simulink model "dc_microgrid_vreg"  (R2015a)
settings: Solver=ode45  StartTime=0.0  StopTime=0.01  RelTol=1e-3
values from neighbouring files (symbols this model uses):
  A = 25*[0 1;1 0]    [parameters_dcmicrogrid.m]    (also in parameters_dcmicrogrid_hynger.m; pendulum_init.m = [0 1 0 0)
  a1v1 = Pmc*a1xpi1    [parameters_dcmicrogrid.m]    (also in parameters_dcmicrogrid_hynger.m)
  a1v2 = Pmc*a1xpi2    [parameters_dcmicrogrid.m]    (also in parameters_dcmicrogrid_hynger.m)
  a1xmc1 = a3    [parameters_dcmicrogrid.m]    (also in parameters_dcmicrogrid_hynger.m)
  a1xmc2 = a3    [parameters_dcmicrogrid.m]    (also in parameters_dcmicrogrid_hynger.m)
  a1xpi1 = Imc*c3    [parameters_dcmicrogrid.m]    (also in parameters_dcmicrogrid_hynger.m)
  a1xpi2 = Imc*c3    [parameters_dcmicrogrid.m]    (also in parameters_dcmicrogrid_hynger.m)
  a2v1 = Pmc*a2xpi1    [parameters_dcmicrogrid.m]    (also in parameters_dcmicrogrid_hynger.m)
  a2v2 = Pmc*a2xpi2    [parameters_dcmicrogrid.m]    (also in parameters_dcmicrogrid_hynger.m)
  a2xmc1 = C(1,2)*P(1,1)*c1/Imax(1)    [parameters_dcmicrogrid.m]    (also in parameters_dcmicrogrid_hynger.m)
  a2xmc2 = C(2,1)*P(2,2)*c1/Imax(2)    [parameters_dcmicrogrid.m]    (also in parameters_dcmicrogrid_hynger.m)
  a2xpi1 = Imc*c2    [parameters_dcmicrogrid.m]    (also in parameters_dcmicrogrid_hynger.m)
  a2xpi2 = Imc*c2    [parameters_dcmicrogrid.m]    (also in parameters_dcmicrogrid_hynger.m)
  a3xmc1 = C(1,2)*P(1,1)*c1/Imax(1) + RD(1,1)*c1    [parameters_dcmicrogrid.m]    (also in parameters_dcmicrogrid_hynger.m)
  a3xmc2 = C(1,2)*P(2,2)*c1/Imax(2) + RD(2,2)*c1    [parameters_dcmicrogrid.m]    (also in parameters_dcmicrogrid_hynger.m)
  axi1 = C(1,2)*I(1,1)*c1/Imax(1)    [parameters_dcmicrogrid.m]    (also in parameters_dcmicrogrid_hynger.m)
  axi2 = C(2,1)*I(2,2)*c1/Imax(2)    [parameters_dcmicrogrid.m]    (also in parameters_dcmicrogrid_hynger.m)
  B = 1*A    [parameters_dcmicrogrid.m]    (also in parameters_dcmicrogrid_hynger.m; pendulum_init.m = [0 ; 1.94 ; 0 ; -4.44 ])
  b2 = 1.94    [pendulum_init.m]
  C1 = 2.2e-3    (= 0.0022)    [parameters_dcmicrogrid.m]    (also in parameters_dcmicrogrid_hynger.m)
  C2 = 2.2e-3    (= 0.0022)    [parameters_dcmicrogrid.m]    (also in parameters_dcmicrogrid_hynger.m)
  I = 3*[1 0; 0 1]    [parameters_dcmicrogrid.m]    (also in parameters_dcmicrogrid_hynger.m)
  iL1_0 = 3.2    [parameters_dcmicrogrid_hynger.m]
  iL2_0 = 3.2    [parameters_dcmicrogrid_hynger.m]
  K = [1 0; 0 2]    [parameters_dcmicrogrid_hynger.m]    (also in pendulum_init.m = K_lmi)
  L1 = 2.65e-3    (= 0.00265)    [parameters_dcmicrogrid.m]    (also in parameters_dcmicrogrid_hynger.m)
  L2 = 2.65e-3    (= 0.00265)    [parameters_dcmicrogrid.m]    (also in parameters_dcmicrogrid_hynger.m)
  P = 0.05*[1 0; 0 1]    [parameters_dcmicrogrid.m]    (also in parameters_dcmicrogrid_hynger.m; pendulum_init.m = [p11 p12 p13 p14; p12 p22 p23 p24; p13 p23 p33 p34; p14 p24 )
  R1 = 20    [parameters_dcmicrogrid.m]    (also in parameters_dcmicrogrid_hynger.m = 30)
  R2 = 20    [parameters_dcmicrogrid.m]    (also in parameters_dcmicrogrid_hynger.m = 30)
  Req = R1*R2/(R1+R2)    (= 10)    [parameters_dcmicrogrid.m]    (also in parameters_dcmicrogrid_hynger.m = 15)
  rL1 = 520e-3    (= 0.52)    [parameters_dcmicrogrid.m]    (also in parameters_dcmicrogrid_hynger.m)
  rL2 = 520e-3    (= 0.52)    [parameters_dcmicrogrid.m]    (also in parameters_dcmicrogrid_hynger.m)
  rs1 = 200e-3    (= 0.2)    [parameters_dcmicrogrid.m]    (also in parameters_dcmicrogrid_hynger.m)
  rs2 = 200e-3    (= 0.2)    [parameters_dcmicrogrid.m]    (also in parameters_dcmicrogrid_hynger.m)
  T1 = 1/60000    (= 1.66666666667e-05)    [parameters_dcmicrogrid.m]    (also in parameters_dcmicrogrid_hynger.m = 6.66666666667e-05)
  T2 = 1/60000    (= 1.66666666667e-05)    [parameters_dcmicrogrid.m]    (also in parameters_dcmicrogrid_hynger.m = 6.66666666667e-05)
  t_0 = 0    [parameters_dcmicrogrid_hynger.m]
  vavgi1_0 = 0    [parameters_dcmicrogrid_hynger.m]
  vavgi2_0 = 0    [parameters_dcmicrogrid_hynger.m]
  vC1_0 = 48.02    [parameters_dcmicrogrid_hynger.m]
  vC2_0 = 48.02    [parameters_dcmicrogrid_hynger.m]
  vesti1_0 = 48.02    [parameters_dcmicrogrid_hynger.m]
  vesti2_0 = 48.02    [parameters_dcmicrogrid_hynger.m]
  Vin1 = Vin(1)    [parameters_dcmicrogrid.m]    (also in parameters_dcmicrogrid_hynger.m)
  Vin2 = Vin(2)    [parameters_dcmicrogrid.m]    (also in parameters_dcmicrogrid_hynger.m)
  Vref1 = Vref(1)    [parameters_dcmicrogrid.m]    (also in parameters_dcmicrogrid_hynger.m)
  Vref2 = Vref(2)    [parameters_dcmicrogrid.m]    (also in parameters_dcmicrogrid_hynger.m)
  westi1_0 = 0    [parameters_dcmicrogrid_hynger.m]
  westi2_0 = 0    [parameters_dcmicrogrid_hynger.m]
  westii1_0 = 0    [parameters_dcmicrogrid_hynger.m]
  westii2_0 = 0    [parameters_dcmicrogrid_hynger.m]
  xi1_0 = 0.01915    [parameters_dcmicrogrid_hynger.m]
  xi2_0 = 0.01915    [parameters_dcmicrogrid_hynger.m]
  xmc1_0 = 2.401    [parameters_dcmicrogrid_hynger.m]
  xmc2_0 = 2.401    [parameters_dcmicrogrid_hynger.m]
  xpi1_0 = 0.51    [parameters_dcmicrogrid_hynger.m]
  xpi2_0 = 0.51    [parameters_dcmicrogrid_hynger.m]
  xpu1_0 = 0.008491    [parameters_dcmicrogrid_hynger.m]
  xpu2_0 = 0.008491    [parameters_dcmicrogrid_hynger.m]
  xvo1_0 = 0.0103    [parameters_dcmicrogrid_hynger.m]
  xvo2_0 = 0.0103    [parameters_dcmicrogrid_hynger.m]
undefined symbols (not defined in the file or in its folder): a1, a2, b1, c1, c2, d1, d2
settings Model: CovSFcnEnable=off  Creator=OmarAli  LastModifiedBy=omar
settings DataIOCC: LimitDataPoints=off
settings DebuggingCC: SolverPrmCheckMsg=warning

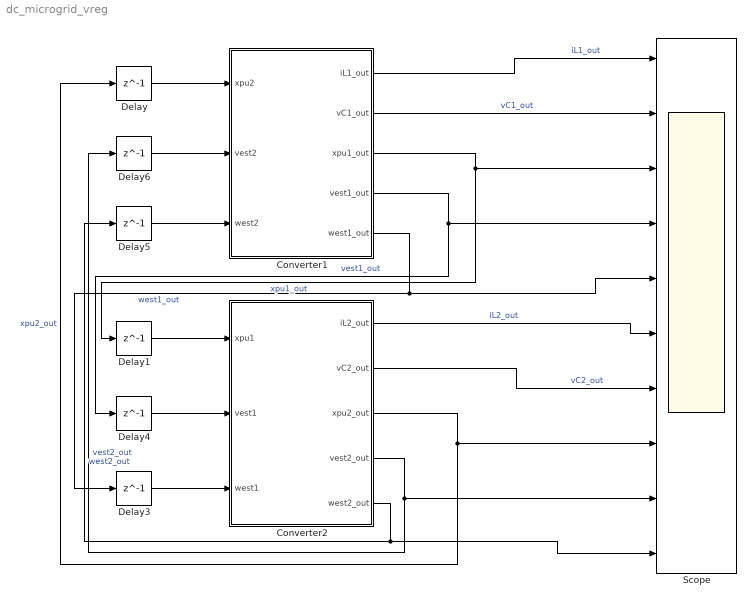
== system dc_microgrid_vreg ==
  Converter1 : Stateflow chart  TreatAsAtomicUnit=on
  Converter2 : Stateflow chart  TreatAsAtomicUnit=on
  Delay{,1,3..6} (6 alike) : Delay  DelayLength=1  InitialCondition=0  SampleTime=1/60000
  Scope : Scope  NumInputPorts=10
      settings: ShowLegends=on  YMin=0~0~0~0~-0.0125~0~0~0~0~-0.0125  YMax=2.5~20~0.0075~20~0.0025~2.5~20~0.0075~20~0.0025
  wires:
  Converter1/3(xpu1_out) -> Scope/3, Delay1/1  "xpu1_out"
  Converter2/3(xpu2_out) -> Scope/8, Delay/1  "xpu2_out"
  Delay/1 -> Converter1/1(xpu2)
  Delay1/1 -> Converter2/1(xpu1)
  Converter1/1(iL1_out) -> Scope/1  "iL1_out"
  Converter1/2(vC1_out) -> Scope/2  "vC1_out"
  Delay4/1 -> Converter2/2(vest1)
  Delay3/1 -> Converter2/3(west1)
  Delay6/1 -> Converter1/2(vest2)
  Delay5/1 -> Converter1/3(west2)
  Converter2/5(west2_out) -> Scope/10, Delay5/1  "west2_out"
  Converter2/4(vest2_out) -> Scope/9, Delay6/1  "vest2_out"
  Converter1/4(vest1_out) -> Scope/4, Delay4/1  "vest1_out"
  Converter1/5(west1_out) -> Delay3/1, Scope/5  "west1_out"
  Converter2/1(iL2_out) -> Scope/6  "iL2_out"
  Converter2/2(vC2_out) -> Scope/7  "vC2_out"

== stateflow chart dc_microgrid_vreg/Converter2 ==
  settings: updateMethod=CONTINUOUS
  state close2
    du:
    iL2_dot = (1/L2)*(-1*(rs2+rL2)*iL2+Vin2 - vC2);
    vC2_dot = (1/C2)*(iL2 - vC2/R2);
    xpu2_dot = a1*xpu2 + b1*iL2;
    xi2_dot = axi2*(xpu1 - xpu2);
    xmc2_dot = a1xmc2*xmc2 + a2xmc2*xpu1 - a3xmc2*xpu2 + xi2+ Vref2+ vavgi2 + (Vref2 - vesti2 - a2xpi2*xvo2 + westii2*K(2,2))*P(2,2);
    xvo2_dot = a2*xvo2 + b2*vC2;
    xpi2_dot = a1xpi2*xmc2 - a2xpi2*xvo2;
    vesti2_dot = (vest1 - vesti2 - a2xpi2*xvo2+ westii2*K(2,2))*A(2,1);
    westi2_dot = (west1 - vesti2 + westii2*K(2,2) - westi2)*B(2,1);
    westii2_dot = vesti2 - westii2*K(2,2) + westi2;
    vavgi2_dot = (Vref2 - vesti2 -  a2xpi2*xvo2 +westii2*K(2,2))*I(2,2);
    t_dot = 1;
    iL2_out = iL2;
    vC2_out = vC2;
    xpu2_out = xpu2;
    vest2_out = vesti2 + a2xpi2*xvo2 - westii2*K(2,2);
    west2_out = westi2 + vesti2 - westii2*K(2,2);
  state open2
    du:
    iL2_dot = (1/L2)*(-rL2*iL2 - vC2);
    vC2_dot = (1/C2)*(iL2 - vC2/R2);
    xpu2_dot = a1*xpu2 + b1*iL2;
    xi2_dot = axi2*(xpu1 - xpu2);
    xmc2_dot = a1xmc2*xmc2 + a2xmc2*xpu1 - a3xmc2*xpu2 + xi2+ Vref2+ vavgi2 + (Vref2 - vesti2 - a2xpi2*xvo2 + westii2*K(2,2))*P(2,2);
    xvo2_dot = a2*xvo2 + b2*vC2;
    xpi2_dot = a1xpi2*xmc2 - a2xpi2*xvo2;
    vesti2_dot = (vest1 - vesti2 - a2xpi2*xvo2+ westii2*K(2,2))*A(2,1);
    westi2_dot = (west1 - vesti2 + westii2*K(2,2) - westi2)*B(2,1);
    westii2_dot = vesti2 - westii2*K(2,2) + westi2;
    vavgi2_dot = (Vref2 - vesti2 -  a2xpi2*xvo2 +westii2*K(2,2))*I(2,2);
    t_dot = 1;
    iL2_out = iL2;
    vC2_out = vC2;
    xpu2_out = xpu2;
    vest2_out = vesti2 + a2xpi2*xvo2 - westii2*K(2,2);
    west2_out = westi2 + vesti2 - westii2*K(2,2);
  state dcm2
    du:
    iL2_dot = 0;
    vC2_dot = - vC2/(R2*C2);
    xpu2_dot = a1*xpu2 + b1*iL2;
    xi2_dot = axi2*(xpu1 - xpu2);
    xmc2_dot = a1xmc2*xmc2 + a2xmc2*xpu1 - a3xmc2*xpu2 + xi2+ Vref2+ vavgi2 + (Vref2 - vesti2 - a2xpi2*xvo2 + westii2*K(2,2))*P(2,2);
    xvo2_dot = a2*xvo2 + b2*vC2;
    xpi2_dot = a1xpi2*xmc2 - a2xpi2*xvo2;
    vesti2_dot = (vest1 - vesti2 - a2xpi2*xvo2+ westii2*K(2,2))*A(2,1);
    westi2_dot = (west1 - vesti2 + westii2*K(2,2) - westi2)*B(2,1);
    westii2_dot = vesti2 - westii2*K(2,2) + westi2;
    vavgi2_dot = (Vref2 - vesti2 -  a2xpi2*xvo2 +westii2*K(2,2))*I(2,2);
    t_dot = 1;
    iL2_out = iL2;
    vC2_out = vC2;
    xpu2_out = xpu2;
    vest2_out = vesti2 + a2xpi2*xvo2 - westii2*K(2,2);
    west2_out = westi2 + vesti2 - westii2*K(2,2);
  close2 -> open2 : [(a1v2*xmc2 - a2v2*xvo2 + xpi2) -  t/T2<= 0]
  (default) -> close2 : {iL2 = iL2_0;
      | vC2 = vC2_0;
      | xpu2 = xpu2_0;
      | xi2 = xi2_0;
      | xmc2 = xmc2_0;
      | xvo2 = xvo2_0;
      | xpi2 = xpi2_0;
      | vesti2 = vesti2_0;
      | westi2 = westi2_0;
      | westii2 = westii2_0;
      | vavgi2 = vavgi2_0;
      | t = t_0;}
  open2 -> close2 [order 2] : [t >= T2]
      | {t = 0;}
  open2 -> dcm2 [order 1] : [iL2 <= 0]
  dcm2 -> close2 : [t >= T2]
      | {t = 0;}
  data: rs2 parameter double; Vref2 parameter double; Vin2 parameter double; rL2 parameter double; iL2_out output double; t local; iL2 local; vC2 local; xi2 local; xvo2 local; xpu2 local; xmc2 local; xpi2 local; T2 parameter double; L2 parameter double; C2 parameter double; R2 parameter double; vC2_out output double; xpu2_out output double; xpu1 input double; a1 parameter double; a2 parameter double; b1 parameter double; b2 parameter double; c1 parameter double; c2 parameter double; d1 parameter double; d2 parameter double; axi2 parameter double; a1xmc2 parameter double; a2xmc2 parameter double; a3xmc2 parameter double; a1xpi2 parameter double; a2xpi2 parameter double; a1v2 parameter double; a2v2 parameter double; Req parameter double; iL2_0 parameter; t_0 parameter; xpu2_0 parameter; xmc2_0 parameter; xvo2_0 parameter; xpi2_0 parameter; vC2_0 parameter; xi2_0 parameter; vest1 input double; west1 input double; vesti2_0 parameter; westi2_0 parameter; westii2_0 parameter; vavgi2_0 parameter; vest2_out output; west2_out output; westi2 local; vavgi2 local; vesti2 local; westii2 local; B parameter; I parameter; A parameter; P parameter; K parameter
  data t settings: updateMethod=SF_CONTINUOUS_TIME_DATA
  data iL2 settings: updateMethod=SF_CONTINUOUS_TIME_DATA
  data vC2 settings: updateMethod=SF_CONTINUOUS_TIME_DATA
  data xi2 settings: updateMethod=SF_CONTINUOUS_TIME_DATA
  data xvo2 settings: updateMethod=SF_CONTINUOUS_TIME_DATA
  data xpu2 settings: updateMethod=SF_CONTINUOUS_TIME_DATA
  data xmc2 settings: updateMethod=SF_CONTINUOUS_TIME_DATA
  data xpi2 settings: updateMethod=SF_CONTINUOUS_TIME_DATA
  data westi2 settings: updateMethod=SF_CONTINUOUS_TIME_DATA
  data vavgi2 settings: updateMethod=SF_CONTINUOUS_TIME_DATA
  data vesti2 settings: updateMethod=SF_CONTINUOUS_TIME_DATA
  data westii2 settings: updateMethod=SF_CONTINUOUS_TIME_DATA

== stateflow chart dc_microgrid_vreg/Converter1 ==
  settings: updateMethod=CONTINUOUS
  state open1
    du:
    iL1_dot = (1/L1)*(-rL1*iL1 - vC1);
    vC1_dot = (1/C1)*(iL1 - vC1/R1);
    xpu1_dot = a1*xpu1 + b1*iL1;
    xi1_dot = axi1*(xpu2 - xpu1);
    xmc1_dot = a1xmc1*xmc1 + a2xmc1*xpu2  - a3xmc1*xpu1 + xi1+ Vref1+ vavgi1 + (Vref1 - vesti1 - a2xpi1*xvo1 + westii1*K(1,1))*P(1,1);
    xvo1_dot = a2*xvo1 + b2*vC1;
    xpi1_dot = a1xpi1*xmc1 - a2xpi1*xvo1;
    vesti1_dot = (vest2 - vesti1 - a2xpi1*xvo1+ westii1*K(1,1))*A(1,2);
    westi1_dot = (west2 - vesti1 + westii1*K(1,1) - westi1)*B(1,2);
    westii1_dot = vesti1 - westii1*K(1,1) + westi1;
    vavgi1_dot = (Vref1 - vesti1 -  a2xpi1*xvo1 +westii1*K(1,1))*I(1,1);
    t_dot = 1;
    iL1_out = iL1;
    vC1_out = vC1;
    xpu1_out = xpu1;
    vest1_out = vesti1 + a2xpi1*xvo1 - westii1*K(1,1);
    west1_out = westi1 + vesti1 - westii1*K(1,1);
  state close1
    du:
    iL1_dot = (1/L1)*(-1*(rs1+rL1)*iL1+Vin1 - vC1);
    vC1_dot = (1/C1)*(iL1 - vC1/R1);
    xpu1_dot = a1*xpu1 + b1*iL1;
    xi1_dot = axi1*(xpu2 - xpu1);
    xmc1_dot = a1xmc1*xmc1 + a2xmc1*xpu2  - a3xmc1*xpu1 + xi1+ Vref1+ vavgi1 + (Vref1 - vesti1 - a2xpi1*xvo1 + westii1*K(1,1))*P(1,1);
    xvo1_dot = a2*xvo1 + b2*vC1;
    xpi1_dot = a1xpi1*xmc1 - a2xpi1*xvo1;
    vesti1_dot = (vest2 - vesti1 - a2xpi1*xvo1+ westii1*K(1,1))*A(1,2);
    westi1_dot = (west2 - vesti1 + westii1*K(1,1) - westi1)*B(1,2);
    westii1_dot = vesti1 - westii1*K(1,1) + westi1;
    vavgi1_dot = (Vref1 - vesti1 -  a2xpi1*xvo1 +westii1*K(1,1))*I(1,1);
    t_dot = 1;
    iL1_out = iL1;
    vC1_out = vC1;
    xpu1_out = xpu1;
    vest1_out = vesti1 + a2xpi1*xvo1 - westii1*K(1,1);
    west1_out = westi1 + vesti1 - westii1*K(1,1);
  state dcm1
    du:
    iL1_dot = 0;
    vC1_dot = - vC1/(R1*C1);
    xpu1_dot = a1*xpu1 + b1*iL1;
    xi1_dot = axi1*(xpu2 - xpu1);
    xmc1_dot = a1xmc1*xmc1 + a2xmc1*xpu2  - a3xmc1*xpu1 + xi1+ Vref1+ vavgi1 + (Vref1 - vesti1 - a2xpi1*xvo1 + westii1*K(1,1))*P(1,1);
    xvo1_dot = a2*xvo1 + b2*vC1;
    xpi1_dot = a1xpi1*xmc1 - a2xpi1*xvo1;
    vesti1_dot = (vest2 - vesti1 - a2xpi1*xvo1+ westii1*K(1,1))*A(1,2);
    westi1_dot = (west2 - vesti1 + westii1*K(1,1) - westi1)*B(1,2);
    westii1_dot = vesti1 - westii1*K(1,1) + westi1;
    vavgi1_dot = (Vref1 - vesti1 -  a2xpi1*xvo1 +westii1*K(1,1))*I(1,1);
    t_dot = 1;
    iL1_out = iL1;
    vC1_out = vC1;
    xpu1_out = xpu1;
    vest1_out = vesti1 + a2xpi1*xvo1 - westii1*K(1,1);
    west1_out = westi1 + vesti1 - westii1*K(1,1);
  close1 -> open1 : [(a1v1*xmc1 - a2v1*xvo1 + xpi1) -  t/T1 <= 0]
  (default) -> close1 : {iL1 = iL1_0;
      | vC1 = vC1_0;
      | xpu1 = xpu1_0;
      | xi1 = xi1_0;
      | xmc1 = xmc1_0;
      | xvo1 = xvo1_0;
      | xpi1 = xpi1_0;
      | vesti1 = vesti1_0;
      | westi1 = westi1_0;
      | westii1 = westii1_0;
      | vavgi1 = vavgi1_0;
      | t = t_0;}
  open1 -> close1 [order 2] : [t >= T1]
      | {t = 0;}
  dcm1 -> close1 : [t >= T1]
      | {t = 0;}
  open1 -> dcm1 [order 1] : [iL1 <= 0]
  data: rL1 parameter double; Vin1 parameter double; rs1 parameter double; Vref1 parameter double; iL1_out output double; xpu1 local; iL1 local; xmc1 local; vC1 local; xpi1 local; xvo1 local; xi1 local; t local; C1 parameter double; R1 parameter double; L1 parameter double; T1 parameter double; vC1_out output double; xpu1_out output double; xpu2 input double; a1 parameter double; a2 parameter double; b1 parameter double; b2 parameter double; c1 parameter double; c2 parameter double; d1 parameter double; d2 parameter double; axi1 parameter double; a1xmc1 parameter double; a2xmc1 parameter double; a3xmc1 parameter double; a1xpi1 parameter double; a2xpi1 parameter double; a1v1 parameter double; a2v1 parameter double; Req parameter double; xvo1_0 parameter; xpi1_0 parameter; xmc1_0 parameter; xi1_0 parameter; iL1_0 parameter; vC1_0 parameter; xpu1_0 parameter; t_0 parameter; vest2 input double; west2 input double; vesti1_0 parameter; westi1_0 parameter; westii1_0 parameter; vavgi1_0 parameter; vest1_out output; west1_out output; vavgi1 local; vesti1 local; westii1 local; westi1 local; K parameter; B parameter; P parameter; A parameter; I parameter
  data xpu1 settings: updateMethod=SF_CONTINUOUS_TIME_DATA
  data iL1 settings: updateMethod=SF_CONTINUOUS_TIME_DATA
  data xmc1 settings: updateMethod=SF_CONTINUOUS_TIME_DATA
  data vC1 settings: updateMethod=SF_CONTINUOUS_TIME_DATA
  data xpi1 settings: updateMethod=SF_CONTINUOUS_TIME_DATA
  data xvo1 settings: updateMethod=SF_CONTINUOUS_TIME_DATA
  data xi1 settings: updateMethod=SF_CONTINUOUS_TIME_DATA
  data t settings: updateMethod=SF_CONTINUOUS_TIME_DATA
  data vavgi1 settings: updateMethod=SF_CONTINUOUS_TIME_DATA
  data vesti1 settings: updateMethod=SF_CONTINUOUS_TIME_DATA
  data westii1 settings: updateMethod=SF_CONTINUOUS_TIME_DATA
  data westi1 settings: updateMethod=SF_CONTINUOUS_TIME_DATA
